simulink model "compensacion_e_integrador"  (R2017a)
settings: Solver=ode45  StartTime=0.0  StopTime=4  RelTol=1e-3  EnableMultiTasking=on
settings Model: Creator=Javi  LastModifiedBy=juanm
settings DataIOCC: LimitDataPoints=on  SaveFormat=Array
settings OptimizationCC: LifeSpan=inf
settings DebuggingCC: SolverPrmCheckMsg=warning  SFUnexpectedBacktrackingDiag=warning  SFNoUnconditionalDefaultTransitionDiag=warning  SFExecutionAtInitializationDiag=none
settings HardwareCC: ProdBitPerPointer=32  ProdBitPerSizeT=32  ProdBitPerPtrDiffT=32  ProdLargestAtomicFloat=None  ProdIntDivRoundTo=Undefined  ProdEndianess=Unspecified  ProdWordSize=32  ProdHWDeviceType=32-bit Generic
settings ModelReferenceCC: PropagateSignalLabelsOutOfModel=off
settings GRTTargetCC: TargetLangStandard=C89/C90 (ANSI)  GeneratePreprocessorConditionals=Disable all
settings ConfigComp: CovMetricSettings=dw  CovHtmlReporting=on  CovSaveCumulativeToWorkspaceVar=on  CovSaveSingleToWorkspaceVar=on  CovExternalEMLEnable=off  CovSFcnEnable=off

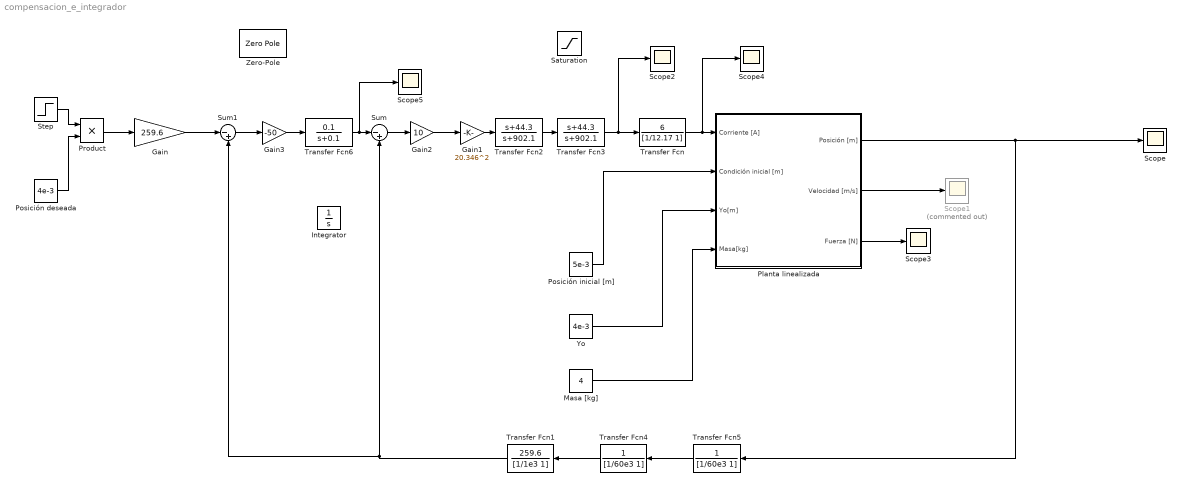
== system compensacion_e_integrador ==
  Gain : Gain  Gain=259.6
  Gain1 : Gain  Gain=20.346^2
  Gain2 : Gain  Gain=10
  Gain3 : Gain  Gain=-50
  Integrator : Integrator
  "Masa [kg] " : Constant  Value=4
  Planta linealizada : Subsystem
  Posición deseada : Constant  Value=4e-3
  "Posición inicial [m] " : Constant  Value=5e-3
  Product : Product
  Saturation : Saturate  UpperLimit=5  LowerLimit=-inf
  Scope{,2..5} (5 alike) : Scope
  Scope1 : Scope  Commented=on
  Step : Step  Time=0.01  SampleTime=0
  Sum : Sum  Inputs=|-+
  Sum1 : Sum  Inputs=|-+
  Transfer Fcn : TransferFcn  Numerator=[6]  Denominator=[1/12.17 1]
  Transfer Fcn1 : TransferFcn  Numerator=259.6  Denominator=[1/1e3 1]
  Transfer Fcn2 : TransferFcn  Numerator=[1 44.3]  Denominator=[1 902.1]
  Transfer Fcn3 : TransferFcn  Numerator=[1 44.3]  Denominator=[1 902.1]
  Transfer Fcn4 : TransferFcn  Numerator=1  Denominator=[1/60e3 1]
  Transfer Fcn5 : TransferFcn  Numerator=1  Denominator=[1/60e3 1]
  Transfer Fcn6 : TransferFcn  Numerator=[0.1]  Denominator=[1 0.1]
  "Yo " : Constant  Value=4e-3
  Zero-Pole : ZeroPole  Zeros=[-221.7 -221.7]  Poles=[-4511 -4511]  Gain=8.28e5
  wires:
  "Posición inicial [m] "/1 -> Planta linealizada/2("Condición inicial [m] ")
  "Yo "/1 -> Planta linealizada/3(Yo[m])
  "Masa [kg] "/1 -> Planta linealizada/4("Masa[kg] ")
  Planta linealizada/1(Posición [m]) -> Transfer Fcn5/1, Scope/1
  Planta linealizada/2(Velocidad [m/s]) -> Scope1/1
  Transfer Fcn1/1 -> Sum1/2, Sum/2
  Transfer Fcn/1 -> Scope4/1, Planta linealizada/1(Corriente [A])
  Planta linealizada/3(Fuerza [N]) -> Scope3/1
  Transfer Fcn3/1 -> Scope2/1, Transfer Fcn/1
  Step/1 -> Product/1
  Posición deseada/1 -> Product/2
  Product/1 -> Gain/1
  Transfer Fcn2/1 -> Transfer Fcn3/1
  Gain1/1 -> Transfer Fcn2/1
  Sum/1 -> Gain2/1
  Gain2/1 -> Gain1/1
  Transfer Fcn4/1 -> Transfer Fcn1/1
  Transfer Fcn5/1 -> Transfer Fcn4/1
  Gain/1 -> Sum1/1
  Sum1/1 -> Gain3/1
  Gain3/1 -> Transfer Fcn6/1
  Transfer Fcn6/1 -> Scope5/1, Sum/1

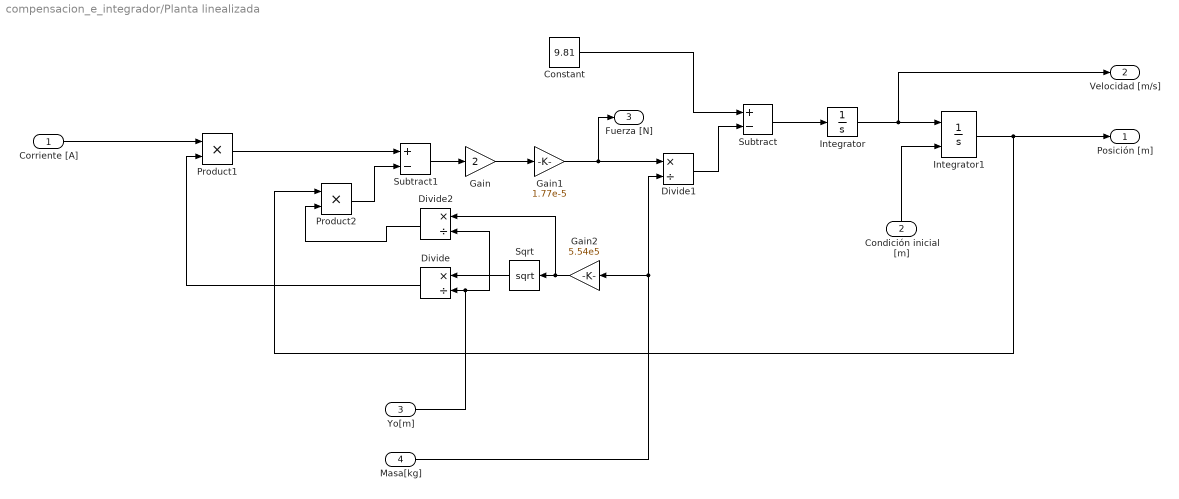
== system compensacion_e_integrador/Planta linealizada ==
  Corriente [A] : Inport
  "Condición inicial [m] " : Inport  Port=2
  Yo[m] : Inport  Port=3
  "Masa[kg] " : Inport  Port=4
  Constant : Constant  Value=9.81
  Divide : Product  Inputs=*/
  Divide1 : Product  Inputs=*/
  Divide2 : Product  Inputs=*/
  Gain : Gain  Gain=2
  Gain1 : Gain  Gain=1.77e-5
  Gain2 : Gain  Gain=5.54e5
  Integrator : Integrator
  Integrator1 : Integrator  InitialConditionSource=external  LimitOutput=on  LowerSaturationLimit=0
  Product1 : Product
  Product2 : Product
  Sqrt : Sqrt  SaturateOnIntegerOverflow=on
  Subtract : Sum  Inputs=+-
  Subtract1 : Sum  Inputs=+-
  Posición [m] : Outport
  Velocidad [m/s] : Outport  Port=2
  Fuerza [N] : Outport  Port=3
  wires:
  Divide1/1 -> Subtract/2
  Gain2/1 -> Divide2/1, Sqrt/1
  Product1/1 -> Subtract1/1
  Corriente [A]/1 -> Product1/1
  Sqrt/1 -> Divide/1
  Yo[m]/1 -> Divide2/2, Divide/2
  Product2/1 -> Subtract1/2
  Divide/1 -> Product1/2
  Divide2/1 -> Product2/2
  "Masa[kg] "/1 -> Gain2/1, Divide1/2
  "Condición inicial [m] "/1 -> Integrator1/2
  Integrator/1 -> Velocidad [m/s]/1, Integrator1/1
  Integrator1/1 -> Posición [m]/1, Product2/1
  Subtract/1 -> Integrator/1
  Subtract1/1 -> Gain/1
  Gain/1 -> Gain1/1
  Gain1/1 -> Fuerza [N]/1, Divide1/1
  Constant/1 -> Subtract/1
